simulink model "req6"  (R2019a)
settings: Solver=FixedStepAuto  StartTime=0.0  StopTime=100  RelTol=1e-3
settings Model: Creator=e40014285  LastModifiedBy=e40014285
settings ConfigComp: CovEnable=on  RecordCoverage=on  CovHtmlReporting=on  CovModelRefEnable=on  DVModelCoverageObjectives=MCDC  DVTestSuiteOptimization=Auto  DVDetectOutOfBounds=on  DVRebuildModelRepresentation=Always

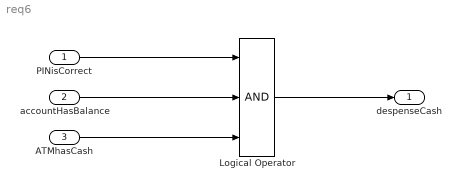
== system req6 ==
  PINisCorrect : Inport  OutDataTypeStr=double
  accountHasBalance : Inport  Port=2  OutDataTypeStr=double
  ATMhasCash : Inport  Port=3  OutDataTypeStr=double
  Logical Operator : Logic  Inputs=3  AllPortsSameDT=off  OutDataTypeStr=boolean
  despenseCash : Outport
  wires:
  Logical Operator/1 -> despenseCash/1
  PINisCorrect/1 -> Logical Operator/1
  accountHasBalance/1 -> Logical Operator/2
  ATMhasCash/1 -> Logical Operator/3
